simulink model "frft_qpsk_transceiver"  (R2025a)
settings: Solver=FixedStepDiscrete  StartTime=0.0  StopTime=1  RelTol=1e-3
PreLoadFcn:
  | % Add paths
  | addpath("dvb-s2/")
  | addpath("frft_filtering/")
  | addpath("gse")
  | 
  | 
  | 
  | 
  | setTxBurstLength = 10000;
  | txtmsg = ['Zynq radio HW/SW Co-design ÞÞÞÞ']; % Use only printable characters
  | 
  | %------------------------------------------------------------------------------------------------------
  | if ~isequal(size(txtmsg),[1 31])
  |     error('txtmsg must contain 31 characters');
  | end
  | 
  | [dataBits,msg] = zynqRadioHWSWQPSKgenHelloworldMsg(20); % generate 20 msgs for LUT
  | msgLUT = uint8(msg);
  | dataBitsLUT = dataBits(:);
  | Rsym                = 25e3;%1.92e6;
  | Config = zynqRadioHWSWQPSKTxRxParameters;
  | fs = Rsym*Config.SamplesPerSymbol;
  | word = [txtmsg newline];  % append a new line character to txtmsg
  | 
  | % The highest clock rate is 16 times the message character rate.
  | % As the message characters are fed at highest clock to FPGA
  | % repeat each character 16 times to maintain the message rate.
  | word = repelem(word.',16,1);
  | repeatTimes = ceil(setTxBurstLength/length(word));
  | inpData = complex(repmat(uint8(word),repeatTimes,1));
  | inUseTxBurstLength = length(inpData);
PostLoadFcn:
  | hScopeConfig = get_param([gcs '/HDL_QPSK/QPSK Tx Channel QPSK Rx/QPSK Rx/Frequency and Time Synchronizer/Symbol Synchronizer/No HDL/QPSK Receiver Eye Diagram'],'ScopeConfiguration');
  | hScopeConfig.OpenAtSimulationStart = false;
  | hScopeConfig.Visible = false;
  | clear hScopeConfig
InitFcn:
  | setTxBurstLength = 10000;
  | txtmsg = ['Zynq radio HW/SW Co-design ÞÞÞÞ']; % Use only printable characters
  | 
  | %------------------------------------------------------------------------------------------------------
  | if ~isequal(size(txtmsg),[1 31])
  |     error('txtmsg must contain 31 characters');
  | end
  | 
  | [dataBits,msg] = zynqRadioHWSWQPSKgenHelloworldMsg(20); % generate 20 msgs for LUT
  | msgLUT = uint8(msg);
  | dataBitsLUT = dataBits(:);
  | Rsym                = 25e3;%1.92e6;
  | Config = zynqRadioHWSWQPSKTxRxParameters;
  | fs = Rsym*Config.SamplesPerSymbol;
  | word = [txtmsg newline];  % append a new line character to txtmsg
  | 
  | % The highest clock rate is 16 times the message character rate.
  | % As the message characters are fed at highest clock to FPGA
  | % repeat each character 16 times to maintain the message rate.
  | word = repelem(word.',16,1);
  | repeatTimes = ceil(setTxBurstLength/length(word));
  | inpData = complex(repmat(uint8(word),repeatTimes,1));
  | inUseTxBurstLength = length(inpData);
undefined symbols (not defined in the file or in its folder): Add, dspblkCoreblockFVToolHelper, gcbh, Shift, unicode2native
libraries: hdlsllib x120, simulink x39, commseqgen3 x8, dsphdlsigops2 x4, whdledac x4, dsphdlfiltering2 x3, whdlutilities x3, dsphdlxfrm2 x2, dsphdlmathfun2 x2, commdigbbndpm3 x2, commchan3 x1, whdlmod x1
(part 1 of 5)
CloseFcn:
  | clear Config dataBits dataBitsLUT fs h inpData ...
  |         inUseTxBurstLength msg msgLUT repeatTimes ...
  |         Rsym setTxBurstLength simAfterCS simBeforeSS ...
  |         simPeakFind simSyncedPackets simTimingOffset ...
  |         simUserData tout txtmsg word captureASCII
settings Model: DataTypeOverride=Off  SimulationMode=accelerator  Creator=The MathWorks, Inc.  LastModifiedBy=daniel
settings DataIOCC: ReturnWorkspaceOutputs=off
settings OptimizationCC: BlockReduction=off  ConditionallyExecuteInputs=off  DefaultParameterBehavior=Inlined  InheritOutputTypeSmallerThanSingle=on  ReuseModelBlockBuffer=off
settings DebuggingCC: AlgebraicLoopMsg=error  SingleTaskRateTransMsg=error  SubsystemReferenceDiagnosticForUnitTest=warning
settings HardwareCC: ProdBitPerPointer=32.0  ProdBitPerSizeT=32.0  ProdBitPerPtrDiffT=32.0  ProdLargestAtomicFloat=None  ProdIntDivRoundTo=Undefined  ProdEndianess=Unspecified  ProdWordSize=32.0  ProdHWDeviceType=ASIC/FPGA->ASIC/FPGA  TargetBitPerLong=64.0  TargetBitPerPointer=64.0  TargetBitPerSizeT=64.0  TargetBitPerPtrDiffT=64.0  TargetLongLongMode=on  TargetIntDivRoundTo=Zero  TargetEndianess=LittleEndian  TargetWordSize=64.0  TargetHWDeviceType=Custom Processor->MATLAB Host Computer  ProdEqTarget=off
settings RTWCC: GPUComputeCapability=3.5

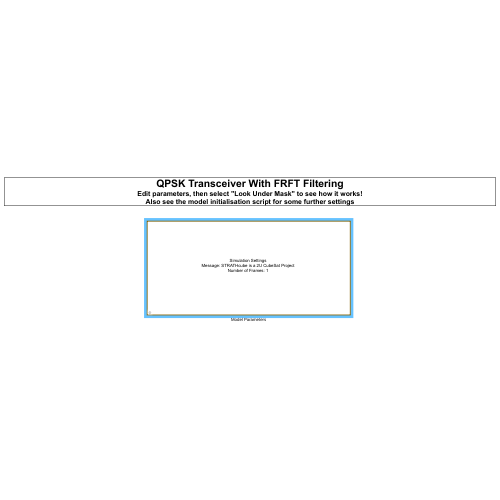
[thumbnail: Simulink's stored preview of the top-level diagram]
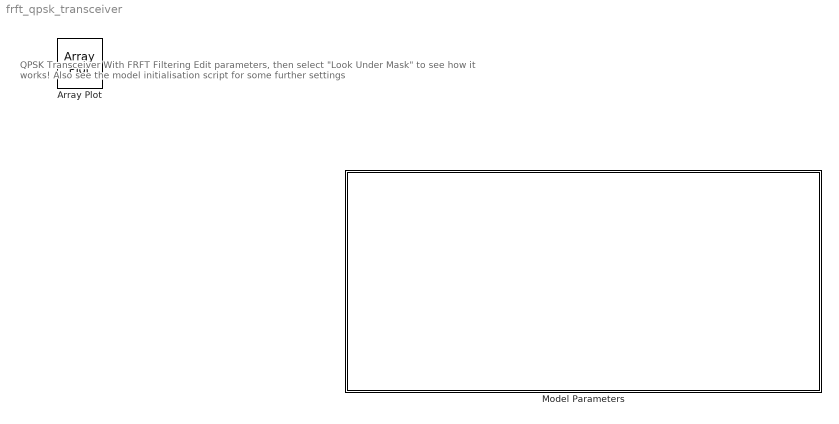
== system frft_qpsk_transceiver ==
  note: QPSK Transceiver With FRFT Filtering
      | Edit parameters, then select "Look Under Mask" to see how it works!
      | Also see the model initialisation script for some further settings
  Model Parameters : Subsystem  mask(Simulation Parameter Controls){fec_en=off, msg="STRATHcube is a 2U CubeSat Project", hmac="SkubeTradeshowDemoKey", n_frames=1, snr=3, interference_en=off, sir=0.1, filter_en=off, altitude=409e3, pass_duration=300, elev_start=10, elev_end=90, fc=435e6}
      mask prompts: fec_en "Enable FEC"; msg "Message Text"; hmac "HMAC Key"; n_frames "N. Frames"; snr "SNR (dB)"; interference_en "Enable Chirp Interference"; sir "SIR (Ratio) (2^n)"; filter_en "Enable Filter"; altitude "Altitude (m)"; pass_duration "Pass Duration (s)"; elev_start "Elevation Start / End (°)"; fc "Carrier Frequency"
      mask help: Sets various parameters for the transceiver system
      mask init:
      | cfg = struct;
      | 
      | % FEC
      | cfg.fec_en = fec_en;
      | gse_frames = gse_genframes(unicode2native(msg),hmac,n_frames)';
      | cfg.FECFRAME = 1120;
      | cfg.DATALENGTH = 840;
      | if fec_en
      |     disp("Using FEC")
      |     
      |     cfg.frames = zeros(cfg.DATALENGTH/8, size(gse_frames,2));
      |     for f = 1:size(gse_frames,2)
      |         frm = gse_frames(:,f);
      |         if length(frm) < cfg.DATALENGTH/8
      |             frm = [frm;zeros(cfg.DATALENGTH/8 - length(frm),1)];
      |         end
      |         cfg.frames(:,f) = frm;
      |     end
      | else
      |     disp("No FEC")
      |     cfg.frames = gse_frames;
      | end
      | 
      | %LDPC Code Setup
      | cfg.parityCheckMatrix =  [5 14 12 1 2 37 45 26 24 0 3 -1 34 7 46 10 -1 -1 -1 -1;
      |     0 35 1 26 0 10 16 16 34 4 2 23 0 51 -1 49 20 -1 -1 -1;
      |     12 28 22 46 3 16 51 2 25 29 19 18 52 -1 37 -1 34 39 -1 -1;
      |     0 51 16 31 13 39 27 33 8 27 53 13 -1 52 33 -1 -1 38 7 -1;
      |     36 6 3 51 4 19 4 45 48 9 -1 11 22 23 43 -1 -1 -1 14 1;];
      | cfg.blockSize = 56;
      | cfg.ipfrms = repelem(cfg.frames(:), 16);
      | 
      | cfg.frame_length = size(cfg.frames,2);
      | cfg.message = msg;
      | cfg.nframes = n_frames;
      | 
      | % Channel
      | cfg.snr = snr; % AWGN
      | 
      | cfg.interference_en = interference_en;
      | cfg.sir = sir;
      | 
      | % Doppler
      | cfg.pass_duration = pass_duration;
      | cfg.doppler_start = dopplerShiftCircularOrbit(elev_start,altitude,10,fc);
      | cfg.doppler_end = dopplerShiftCircularOrbit(elev_end,altitude,10,fc);
      | 
      | cfg.filter_en = filter_en;
      mask DialogControl Container6 Prompt: Transmitter
      mask DialogControl ParameterGroupVar Prompt: GSE Protocol
      mask DialogControl Container3 Prompt: Channel
      mask DialogControl Container4 Prompt: Interference
      mask DialogControl Container5 Prompt: Doppler
      mask Display:
      | icon_txt = sprintf( ...
      |     "Simulation Settings \n" + ...
      |     "Message: %s \n"+ ...
      |     "Number of Frames: %i \n", ...
      |     msg, n_frames ...
      |     );
      | 
      | disp(icon_txt);
  Array Plot : ArrayPlot  IOType=viewer  IsFloating=on  WindowPosition=[560.000000,491.000000,800.000000,500.000000,]  Visible=on  ScopeFrameLocation=window  YLimits=[-203.25 399.25]  DefaultConfigurationName=dsp.scopes.ArrayPlotBlockSpecification

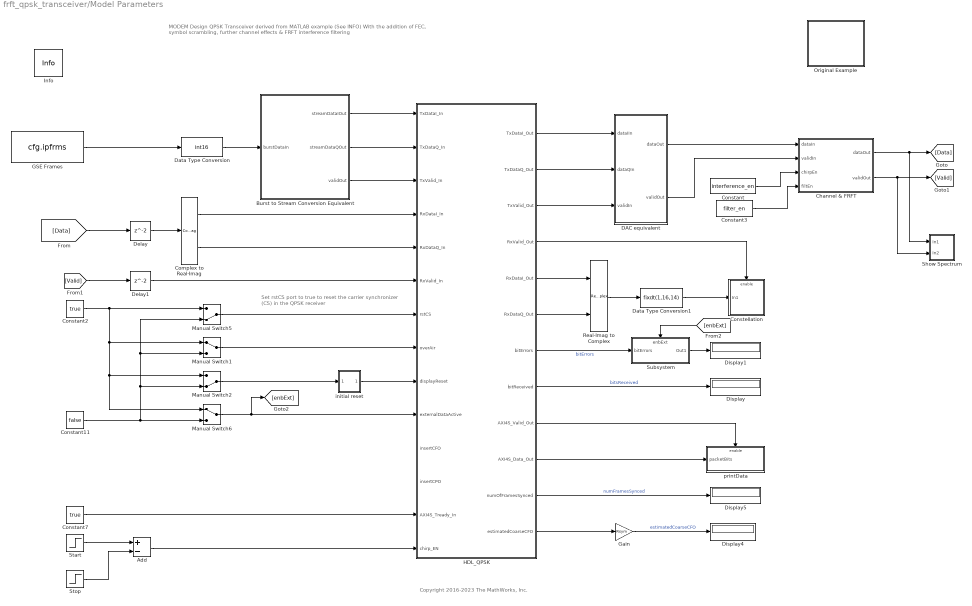
== system frft_qpsk_transceiver/Model Parameters ==
  note: Set rstCS port to true to reset the carrier synchronizer (CS) in the QPSK receiver
  note: Copyright 2016-2023 The MathWorks, Inc.
  note: MODEM Design
      | QPSK Transceiver derived from MATLAB example (See INFO)
      | With the addition of FEC, symbol scrambling, further channel effects & FRFT interference filtering
  Add : Sum  Inputs=+-  OutMin=0  OutMax=1  OutDataTypeStr=fixdt(0,1)
  Burst to Stream Conversion Equivalent : Subsystem
  Channel & FRFT : Subsystem
  Complex to Real-Imag : ComplexToRealImag
  Constant : Constant  Value=interference_en  OutDataTypeStr=boolean
  Constant11 : Constant  Value=false  OutDataTypeStr=boolean  SampleTime=1/fs
  Constant2 : Constant  Value=true  OutDataTypeStr=boolean  SampleTime=1/fs
  Constant3 : Constant  Value=filter_en  OutDataTypeStr=boolean
  Constant7 : Constant  Value=true  OutDataTypeStr=boolean  SampleTime=1/fs
  Constellation : Subsystem
  DAC equivalent : Subsystem
  Data Type Conversion : DataTypeConversion  OutDataTypeStr=int16  SaturateOnIntegerOverflow=off  RndMeth=Floor
  Data Type Conversion1 : DataTypeConversion  OutDataTypeStr=fixdt(1,16,14)  ConvertRealWorld=Stored Integer (SI)  SaturateOnIntegerOverflow=off  RndMeth=Floor
  Delay : Delay
  Delay1 : Delay
  Display{,1,4..5} (4 alike) : Display
  GSE Frames : Constant  Value=cfg.ipfrms  SampleTime=-1
  Gain : Gain  Gain=Rsym  OutDataTypeStr=double
  HDL_QPSK : Subsystem  TreatAsAtomicUnit=on
  Info : sdrzblksprivate/Info  SystemSampleTime=-1  VariantActivationTime=update diagram  EmptyChoice=off  PassThrough=off  PassThroughVariantControl=(default)  EmptyChoiceVariantControl=(default)  AllowFlexibleInterface=on  Latency=0  AutoFrameSizeCalculation=off
  Manual Switch1 : ManualSwitch
  Manual Switch2 : ManualSwitch  CurrentSetting=0
  Manual Switch5 : ManualSwitch  CurrentSetting=0
  Manual Switch6 : ManualSwitch
  Original Example : Subsystem
      settings: OpenFcn="sdrzdoc(\"QPSKTransmitAndReceiveUsingAnalogDevicesAD9361AD9364Example\")"
      mask Display: disp('INFO');
  Real-Imag to Complex : RealImagToComplex
  Show Spectrum : Subsystem
  Start : Step  Time=200e3/fs  SampleTime=1/fs
  Stop : Step  Time=400e3/fs  SampleTime=1/fs
  Subsystem : Subsystem
      settings: PortSchema="{\"entries\":[{\"content\":{\"sides\":[{\"content\":{\"connectorIds\":[\"In1\"]},\"type\":\"ConnectorPlacement.EquallySpacedRectSide\",\"uuid\":\"00e2ba4b-7eac-479c-adca-0b3a47f26300\"},{\"content\":{\"connectorIds\":[\"Out1\"],\"side\":\"RIGHT\"},\"type\":\"ConnectorPlacement.EquallySpacedRectSide\",\"uuid\":\"f46d1850-7aaf-4a4a-a0f0-18f53e4dd1ab\"},{\"content\":{\"connectorIds\":[\"In2\"],\"side\":\"TOP\"},\"type\":\"ConnectorPlacement.EquallySpacedRectSide\",\"uuid\":\"6eb79df9-d0ed-4616-8b56-bf03dd754f89\"}]},\"type\":\"ConnectorPlacement.EquallySpacedConnector\",\"uuid\":\"71623fc3-6fb3-42f9-b5c9-cd74da1aa0dd\"}],\"packageUris\":[\"http://schema.mathworks.com/mf0/Connector/R2020b\"],\"version\":\"1.0\"}"
  initial reset : Subsystem
  printData : Subsystem
  wires:
  initial reset/1(Out1) -> HDL_QPSK/9(displayReset)
  HDL_QPSK/9(AXI4S_Valid_Out) -> printData/Enable
  Burst to Stream Conversion Equivalent/2(streamDataQOut) -> HDL_QPSK/2(TxDataQ_In)
  DAC equivalent/2(validOut) -> Channel & FRFT/2(validIn)
  Add/1 -> HDL_QPSK/14(chirp_EN)
  Constant/1 -> Channel & FRFT/3(chirpEn)
  DAC equivalent/1(dataOut) -> Channel & FRFT/1(dataIn)
  HDL_QPSK/4(RxValid_Out) -> Constellation/Enable
  Start/1 -> Add/1
  Complex to Real-Imag/1 -> HDL_QPSK/4(RxDataI_In)
  HDL_QPSK/8(bitReceived) -> Display/1  "bitsReceived"
  Data Type Conversion/1 -> Burst to Stream Conversion Equivalent/1(burstDataIn)
  Channel & FRFT/1(dataOut) -> Show Spectrum/1(In1), [Data]
  Real-Imag to Complex/1 -> Data Type Conversion1/1
  Subsystem/1(Out1) -> Display1/1
  Constant11/1 -> Manual Switch6/2, Manual Switch5/2, Manual Switch1/2, Manual Switch2/2
  ? -> HDL_QPSK/12(insertCPO)
  [Data] -> Delay/1
  [enbExt] -> Subsystem/2(enbExt)
  Manual Switch1/1 -> HDL_QPSK/8(overAir)
  Data Type Conversion1/1 -> Constellation/1(In1)
  Stop/1 -> Add/2
  Burst to Stream Conversion Equivalent/1(streamDataIOut) -> HDL_QPSK/1(TxDataI_In)
  Constant2/1 -> Manual Switch6/1, Manual Switch2/1, Manual Switch1/1, Manual Switch5/1
  Complex to Real-Imag/2 -> HDL_QPSK/5(RxDataQ_In)
  HDL_QPSK/6(RxDataQ_Out) -> Real-Imag to Complex/2
  HDL_QPSK/1(TxDataI_Out) -> DAC equivalent/1(dataIIn)
  [Valid] -> Delay1/1
  Burst to Stream Conversion Equivalent/3(validOut) -> HDL_QPSK/3(TxValid_In)
  Constant3/1 -> Channel & FRFT/4(filtEn)
  HDL_QPSK/5(RxDataI_Out) -> Real-Imag to Complex/1
  Gain/1 -> Display4/1  "estimatedCoarseCFO"
  Delay1/1 -> HDL_QPSK/6(RxValid_In)
  HDL_QPSK/2(TxDataQ_Out) -> DAC equivalent/2(dataQIn)
  HDL_QPSK/11(numOfFramesSynced) -> Display5/1  "numFramesSynced"
  Manual Switch2/1 -> initial reset/1(In2)
  GSE Frames/1 -> Data Type Conversion/1
  HDL_QPSK/3(TxValid_Out) -> DAC equivalent/3(validIn)
  Constant7/1 -> HDL_QPSK/13(AXI4S_Tready_In)
  HDL_QPSK/10(AXI4S_Data_Out) -> printData/1(packetBits)
  Channel & FRFT/2(validOut) -> Show Spectrum/2(In2), [Valid]
  HDL_QPSK/12(estimatedCoarseCFO) -> Gain/1
  Delay/1 -> Complex to Real-Imag/1
  Manual Switch5/1 -> HDL_QPSK/7(rstCS)
  HDL_QPSK/7(bitErrors) -> Subsystem/1(bitErrors)  "bitErrors"
  Manual Switch6/1 -> HDL_QPSK/10(externalDataActive), [enbExt]

== system frft_qpsk_transceiver/Model Parameters/Burst to Stream Conversion Equivalent ==
  note: The burst data sent from the processing system will be stored in the RAM in the memory channel of SDR IIO radio. The data stored will be poped out as a stream data.
  note: This subsystem does an equivalent operation to simulate the input and output behaviour of the memory channel of the SDR IIO radio.
  burstDataIn : Inport
  Complex to Real-Imag : ComplexToRealImag
  Serializer1D : hdlsllib/HDL Operations/Serializer1D  Ratio=length(cfg.ipfrms)  IdleCycles=0  validIn=off  startOut=off  validOut=on  inputDataDimensions=-1  inputSampleTime=-1  inputSignalType=auto
  streamDataIOut : Outport
  streamDataQOut : Outport  Port=2
  validOut : Outport  Port=3
  wires:
  burstDataIn/1 -> Serializer1D/1
  Serializer1D/1 -> Complex to Real-Imag/1
  Complex to Real-Imag/1 -> streamDataIOut/1
  Complex to Real-Imag/2 -> streamDataQOut/1
  Serializer1D/2 -> validOut/1

== system frft_qpsk_transceiver/Model Parameters/Channel & FRFT ==
  note: Pass through data when chirpEn = 0, otherwise do filtering
  dataIn : Inport
  validIn : Inport  Port=2
  chirpEn : Inport  Port=3
  filtEn : Inport  Port=4
  AWGN : Subsystem
  Data Type Conversion5 : DataTypeConversion  OutDataTypeStr=int16  ConvertRealWorld=Stored Integer (SI)  SaturateOnIntegerOverflow=off  RndMeth=Floor
  Doppler Shift : Subsystem
  Subsystem : Subsystem
  Switch : Switch  Criteria=u2 > Threshold  SaturateOnIntegerOverflow=off  InputSameDT=off
  Switch1 : Switch  Criteria=u2 > Threshold  SaturateOnIntegerOverflow=off  InputSameDT=off
  add_chirp : MATLAB Function  TreatAsAtomicUnit=on  mask{fs=fs, T=32e-3, f0=0, f1=0.9*fs/2, sir=sir}
      mask prompts: sir "SIR (Ratio)"
  dataOut : Outport
      settings: SignalType=complex
  validOut : Outport  Port=2
  wires:
  Switch1/1 -> validOut/1
  chirpEn/1 -> add_chirp/3(chirpEn)
  add_chirp/1(sigOut) -> Switch/3, Subsystem/1(sigIn)  "chirp_sig"
  add_chirp/2(validOut) -> Switch1/3, Subsystem/2(validIn)
  filtEn/1 -> Switch1/2, Switch/2
  Subsystem/2(ValidOut) -> Switch1/1
  Subsystem/1(S) -> Switch/1
  Switch/1 -> Data Type Conversion5/1
  Data Type Conversion5/1 -> dataOut/1
  dataIn/1 -> Doppler Shift/1(dataIn)
  validIn/1 -> Doppler Shift/2(validIn)
  Doppler Shift/1(Out1) -> AWGN/1(dataIn)
  Doppler Shift/2(Out2) -> AWGN/2(validIn)
  AWGN/1(dataOut) -> add_chirp/1(sigIn)
  AWGN/2(validOut) -> add_chirp/2(validIn)

== system frft_qpsk_transceiver/Model Parameters/Constellation ==
  In1 : Inport
  Enable : EnablePort
  Constellation Diagram : ConstellationDiagram  WindowPosition=[1388.000000,624.000000,653.000000,531.000000,]  Visible=on  ScopeFrameLocation=window  SymbolsToDisplaySource=Property  SymbolsToDisplay=10000  XLimits=[-1.38,1.38]  YLimits=[-1.38,1.38]  AxesLimits=[-1.38,1.38]  DefaultConfigurationName=comm.scopes.ConstellationDiagramBlockCfg
  Terminator : Terminator
  wires:
  In1/1 -> Constellation Diagram/1, Terminator/1

== system frft_qpsk_transceiver/Model Parameters/DAC equivalent ==
  dataIIn : Inport
  dataQIn : Inport  Port=2
  validIn : Inport  Port=3
  Data Type Conversion : DataTypeConversion  OutDataTypeStr=int16  SaturateOnIntegerOverflow=off  RndMeth=Floor
  Extract Bits : simulink/Logic and Bit Operations/Extract Bits  bitsToExtract=Range starting with most significant bit  numBits=12  bitIdxRange=[0 7]  outScalingMode=Treat bit field as an integer
  Extract Bits1 : simulink/Logic and Bit Operations/Extract Bits  bitsToExtract=Range starting with most significant bit  numBits=12  bitIdxRange=[0 7]  outScalingMode=Treat bit field as an integer
  Real-Imag to Complex : RealImagToComplex
  dataOut : Outport
  validOut : Outport  Port=2
  wires:
  dataIIn/1 -> Extract Bits/1
  dataQIn/1 -> Extract Bits1/1
  Extract Bits/1 -> Real-Imag to Complex/1
  Extract Bits1/1 -> Real-Imag to Complex/2
  Real-Imag to Complex/1 -> Data Type Conversion/1
  validIn/1 -> validOut/1
  Data Type Conversion/1 -> dataOut/1

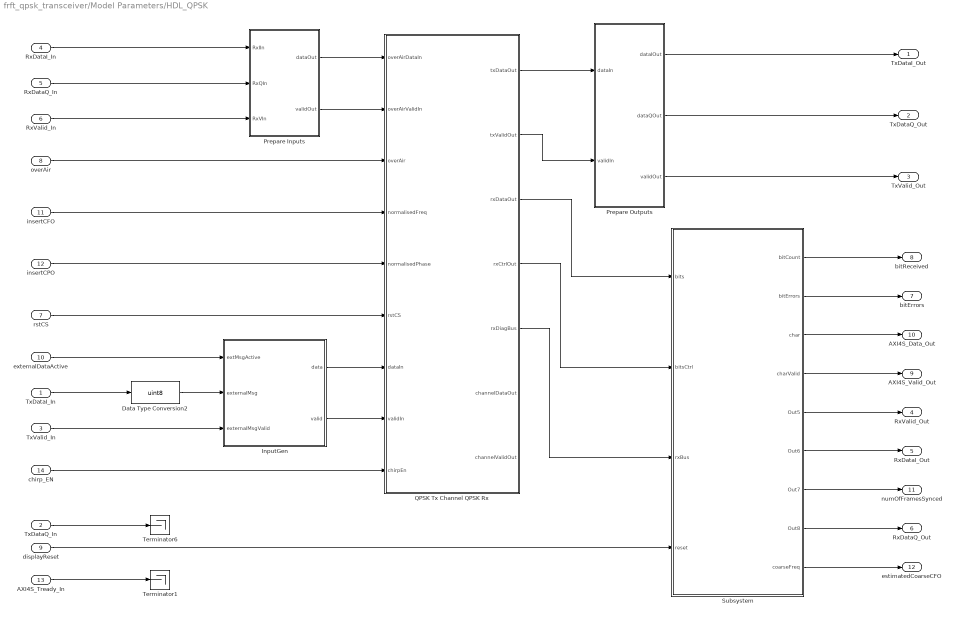
== system frft_qpsk_transceiver/Model Parameters/HDL_QPSK ==
  TxDataI_In : Inport
  TxDataQ_In : Inport  Port=2
  TxValid_In : Inport  Port=3
  RxDataI_In : Inport  Port=4
  RxDataQ_In : Inport  Port=5
  RxValid_In : Inport  Port=6
  rstCS : Inport  Port=7
  overAir : Inport  Port=8
  displayReset : Inport  Port=9
  externalDataActive : Inport  Port=10
  insertCFO : Inport  Port=11
  insertCPO : Inport  Port=12
  AXI4S_Tready_In : Inport  Port=13
  chirp_EN : Inport  Port=14
  Data Type Conversion2 : DataTypeConversion  OutDataTypeStr=uint8  SaturateOnIntegerOverflow=off  RndMeth=Floor
  InputGen : Subsystem
  Prepare Inputs : Subsystem
  Prepare Outputs : Subsystem
  QPSK Tx Channel QPSK Rx : Subsystem
  Subsystem : Subsystem
  Terminator1 : Terminator
  Terminator6 : Terminator
  TxDataI_Out : Outport
  TxDataQ_Out : Outport  Port=2
  TxValid_Out : Outport  Port=3
  RxValid_Out : Outport  Port=4
  RxDataI_Out : Outport  Port=5
  RxDataQ_Out : Outport  Port=6
  bitErrors : Outport  Port=7
  bitReceived : Outport  Port=8
  AXI4S_Valid_Out : Outport  Port=9
  AXI4S_Data_Out : Outport  Port=10
  numOfFramesSynced : Outport  Port=11
  estimatedCoarseCFO : Outport  Port=12
  wires:
  Prepare Outputs/2(dataQOut) -> TxDataQ_Out/1
  Prepare Outputs/3(validOut) -> TxValid_Out/1
  AXI4S_Tready_In/1 -> Terminator1/1
  Prepare Inputs/1(dataOut) -> QPSK Tx Channel QPSK Rx/1(overAirDataIn)
  Prepare Inputs/2(validOut) -> QPSK Tx Channel QPSK Rx/2(overAirValidIn)
  InputGen/1(data) -> QPSK Tx Channel QPSK Rx/7(dataIn)
  InputGen/2(valid) -> QPSK Tx Channel QPSK Rx/8(validIn)
  overAir/1 -> QPSK Tx Channel QPSK Rx/3(overAir)
  insertCFO/1 -> QPSK Tx Channel QPSK Rx/4(normalisedFreq)
  insertCPO/1 -> QPSK Tx Channel QPSK Rx/5(normalisedPhase)
  QPSK Tx Channel QPSK Rx/1(txDataOut) -> Prepare Outputs/1(dataIn)
  QPSK Tx Channel QPSK Rx/2(txValidOut) -> Prepare Outputs/2(validIn)
  displayReset/1 -> Subsystem/4(reset)
  QPSK Tx Channel QPSK Rx/3(rxDataOut) -> Subsystem/1(bits)
  QPSK Tx Channel QPSK Rx/4(rxCtrlOut) -> Subsystem/2(bitsCtrl)
  QPSK Tx Channel QPSK Rx/5(rxDiagBus) -> Subsystem/3(rxBus)
  Subsystem/1(bitCount) -> bitReceived/1
  Subsystem/2(bitErrors) -> bitErrors/1
  Subsystem/3(char) -> AXI4S_Data_Out/1
  Subsystem/4(charValid) -> AXI4S_Valid_Out/1
  Subsystem/5(Out5) -> RxValid_Out/1
  Subsystem/6(Out6) -> RxDataI_Out/1
  Subsystem/7(Out7) -> numOfFramesSynced/1
  Subsystem/8(Out8) -> RxDataQ_Out/1
  rstCS/1 -> QPSK Tx Channel QPSK Rx/6(rstCS)
  Subsystem/9(coarseFreq) -> estimatedCoarseCFO/1
  Prepare Outputs/1(dataIOut) -> TxDataI_Out/1
  RxDataI_In/1 -> Prepare Inputs/1(RxIIn)
  RxDataQ_In/1 -> Prepare Inputs/2(RxQIn)
  RxValid_In/1 -> Prepare Inputs/3(RxVIn)
  TxValid_In/1 -> InputGen/3(externalMsgValid)
  TxDataQ_In/1 -> Terminator6/1
  externalDataActive/1 -> InputGen/1(extMsgActive)
  TxDataI_In/1 -> Data Type Conversion2/1
  Data Type Conversion2/1 -> InputGen/2(externalMsg)
  chirp_EN/1 -> QPSK Tx Channel QPSK Rx/9(chirpEn)

== system frft_qpsk_transceiver/Model Parameters/Original Example ==

== system frft_qpsk_transceiver/Model Parameters/Show Spectrum ==
  In1 : Inport
  In2 : Inport  Port=2
  Compare To Constant : simulink/Logic and Bit Operations/Compare To Constant  relop===  const=inf  OutDataTypeStr=boolean
  Compare To Constant1 : simulink/Logic and Bit Operations/Compare To Constant  relop===  const=NaN  OutDataTypeStr=boolean
  Constant1 : Constant  Value=complex(0+0i)
  Data Type Conversion5 : DataTypeConversion  OutDataTypeStr=double  ConvertRealWorld=Stored Integer (SI)  SaturateOnIntegerOverflow=off  RndMeth=Floor
  Delay2 : Delay  DelayLength=1
  Delay3 : Delay  DelayLength=1
  OR : Logic  Operator=OR  IconShape=distinctive  AllPortsSameDT=off  OutDataTypeStr=boolean
  Spectrum Analyzer : SpectrumAnalyzer  WindowPosition=[511.000000,647.000000,1440.000000,699.000000,]  Visible=on  ScopeFrameLocation=window  ViewType=Spectrum and spectrogram  WindowInvariantSamplesPerUpdate=on  Span=160000  StartFrequency=-80000  StopFrequency=80000  YLimits=[-22.703734811580006 91.64033184798589]  ColorLimits=[NaN NaN]
  Switch : Switch  Criteria=u2 > Threshold  OutDataTypeStr=Inherit: Inherit via back propagation  SaturateOnIntegerOverflow=off
  Switch1 : Switch  Criteria=u2 > Threshold  OutDataTypeStr=Inherit: Inherit via back propagation  SaturateOnIntegerOverflow=off
  wires:
  Delay2/1 -> Delay3/1
  Compare To Constant/1 -> OR/1
  Constant1/1 -> Switch1/1, Switch/3
  Delay3/1 -> Switch1/3
  Data Type Conversion5/1 -> Switch/1
  Switch/1 -> Delay2/1, Compare To Constant1/1, Compare To Constant/1
  Switch1/1 -> Spectrum Analyzer/1
  OR/1 -> Switch1/2
  In2/1 -> Switch/2
  Compare To Constant1/1 -> OR/2
  In1/1 -> Data Type Conversion5/1

== system frft_qpsk_transceiver/Model Parameters/Subsystem ==
  note: 2^32-1 will be treated as NaN in double when converted to double
  bitErrors : Inport
  enbExt : Inport  Port=2
  Compare To Constant : simulink/Logic and Bit Operations/Compare To Constant  relop===  const=2^32-1  OutDataTypeStr=boolean
  Constant : Constant  Value=2^32-1  OutDataTypeStr=uint32  SampleTime=-1
  Constant1 : Constant  Value=NaN  SampleTime=-1
  Data Type Conversion3 : DataTypeConversion  OutDataTypeStr=double  SaturateOnIntegerOverflow=off  RndMeth=Floor
  Switch : Switch  Criteria=u2 ~= 0  SaturateOnIntegerOverflow=off  InputSameDT=off
  Switch1 : Switch  Criteria=u2 ~= 0  SaturateOnIntegerOverflow=off  InputSameDT=off
  Out1 : Outport
  wires:
  Constant/1 -> Switch/1
  bitErrors/1 -> Switch/3
  enbExt/1 -> Switch/2
  Compare To Constant/1 -> Switch1/2
  Switch1/1 -> Out1/1
  Switch/1 -> Data Type Conversion3/1, Compare To Constant/1
  Data Type Conversion3/1 -> Switch1/3
  Constant1/1 -> Switch1/1

== system frft_qpsk_transceiver/Model Parameters/initial reset ==
  In2 : Inport
  Constant : Constant  OutDataTypeStr=boolean  SampleTime=-1
  Delay : Delay  DelayLength=1
  Logical Operator : Logic  Operator=OR  IconShape=distinctive  AllPortsSameDT=off  OutDataTypeStr=boolean
  Logical Operator1 : Logic  Operator=XOR  IconShape=distinctive  AllPortsSameDT=off  OutDataTypeStr=boolean
  Out1 : Outport
  wires:
  In2/1 -> Logical Operator/2
  Logical Operator1/1 -> Logical Operator/1
  Logical Operator/1 -> Out1/1
  Constant/1 -> Delay/1, Logical Operator1/1
  Delay/1 -> Logical Operator1/2

== system frft_qpsk_transceiver/Model Parameters/printData ==
  packetBits : Inport
  Enable : EnablePort  PropagateVarSize=During execution
  Extract Bits : simulink/Logic and Bit Operations/Extract Bits  bitsToExtract=Range ending with least significant bit  numBits=8  bitIdxRange=[0 7]  outScalingMode=Treat bit field as an integer
  Extract Bits1 : simulink/Logic and Bit Operations/Extract Bits  bitsToExtract=Range of bits  numBits=8  bitIdxRange=[8,8]  outScalingMode=Treat bit field as an integer
  Extract Bits2 : simulink/Logic and Bit Operations/Extract Bits  bitsToExtract=Range of bits  numBits=8  bitIdxRange=[9,9]  outScalingMode=Treat bit field as an integer
  MATLAB Function : MATLAB Function  TreatAsAtomicUnit=on  mask{msg_length=size(cfg.frames,1)  - 9 - 32+1, frame_length=size(cfg.frames,1), msg_orig=unicode2native(msg)}
      mask prompts: msg_length "Message Length"; frame_length "Frame Length"; msg_orig "Original Message"
  RxFrame : ToWorkspace  VariableName=RxFrame  SaveFormat=Structure  SampleTime=-1
      settings: Save2DSignal=2-D array (concatenate along first dimension)
  RxFrameValid : ToWorkspace  VariableName=RxFrameValid  SampleTime=-1
      settings: Save2DSignal=2-D array (concatenate along first dimension)
  Serializer1D : hdlsllib/HDL Operations/Serializer1D  Ratio=1  IdleCycles=0  validIn=off  startOut=off  validOut=off  inputDataDimensions=-1  inputSampleTime=-1  inputSignalType=auto
  captureASCII : ToWorkspace  VariableName=captureASCII  SampleTime=-1
      settings: Save2DSignal=2-D array (concatenate along first dimension)
  wires:
  packetBits/1 -> Serializer1D/1
  Serializer1D/1 -> Extract Bits/1, Extract Bits1/1, Extract Bits2/1
  Extract Bits/1 -> MATLAB Function/3(u), captureASCII/1
  Extract Bits2/1 -> MATLAB Function/1(frm_start)
  Extract Bits1/1 -> MATLAB Function/2(frm_end)
  MATLAB Function/1(frameOut) -> RxFrame/1
  MATLAB Function/2(frameValid) -> RxFrameValid/1

== system frft_qpsk_transceiver/Model Parameters/Channel & FRFT/AWGN ==
  dataIn : Inport
  validIn : Inport  Port=2
  AWGN Channel : commchan3/AWGN Channel  LegacyMode=off  NoiseMethod="Signal to noise ratio  (SNR)"  noiseMode="Signal to noise ratio  (SNR)"  EbNo=10  EsNo=10  SNR=cfg.snr-30  BitsPerSymbol=1  SignalPower=1  SpecifySymbolPeriod=off  SamplesPerSymbol=1  SymbolPeriod=1  VarianceSource=Parameter  Variance=1  RandomStream=Global stream  Seed=67  SimulateUsing=Code generation
  Cast : DataTypeConversion  SaturateOnIntegerOverflow=off  RndMeth=Floor
  Delay : Delay  DelayLength=1
  dataOut : Outport
  validOut : Outport  Port=2
  wires:
  Cast/1 -> AWGN Channel/1
  dataIn/1 -> Cast/1  "awgn_in"
  Delay/1 -> validOut/1
  AWGN Channel/1 -> dataOut/1  "awgn_out"
  validIn/1 -> Delay/1

== system frft_qpsk_transceiver/Model Parameters/Channel & FRFT/Doppler Shift ==
  dataIn : Inport
  validIn : Inport  Port=2
  CPO : Constant  Value=fi(phase,1,21,21)  SampleTime=1/fs  mask{phased=0}
      mask prompts: phased "CPO (degrees):"
      mask init:
      | phase = phased/360;
      mask DialogControl DescGroupVar Prompt: Insert CPO
      mask DialogControl DescTextVar Prompt: Introduce CPO into transmitter waveform. The overAir port must be set to false. CPO range: -180 to less than 180
      mask Display: disp(get_param(gcb,"phased"));
  Data Type Conversion : DataTypeConversion  OutDataTypeStr=fixdt(1,21,0)  ConvertRealWorld=Stored Integer (SI)  SaturateOnIntegerOverflow=off  RndMeth=Floor
  Data Type Conversion1 : DataTypeConversion  OutDataTypeStr=fixdt(1,21,0)  ConvertRealWorld=Stored Integer (SI)  SaturateOnIntegerOverflow=off  RndMeth=Floor
  Delay : Delay  DelayLength=6
  Doppler Shift : Sin  SineType=Sample based  Amplitude=-cfg.doppler_start  Frequency=2*pi  Phase=pi  Samples=cfg.pass_duration*fs  SampleTime=1/fs
  NCO HDL Optimized : dsphdlsigops2/NCO  PhaseIncrementSource=Input port  PhaseIncrement=100  PhaseOffsetSource=Input port  PhaseOffset=0  DitherSource=Property  NumDitherBits=11  SamplesPerFrame=1  LUTCompress=off  ResetAction=off  Waveform=Complex exponential  PhasePort=off  SimulateUsing=Code generation  AccumulatorWL=21  PhaseQuantization=on  NumQuantizerAccumulatorBits=14  OutputDataType=Binary point scaling  OutputWL=16  OutputFL=14
  Product : Product  OutDataTypeStr=Inherit: Same as first input
  Out1 : Outport
  Out2 : Outport  Port=2
  wires:
  dataIn/1 -> Delay/1
  Delay/1 -> Product/1
  Data Type Conversion/1 -> NCO HDL Optimized/1
  NCO HDL Optimized/1 -> Product/2
  Product/1 -> Out1/1
  Data Type Conversion1/1 -> NCO HDL Optimized/2
  Doppler Shift/1 -> Data Type Conversion/1
  NCO HDL Optimized/2 -> Out2/1
  CPO/1 -> Data Type Conversion1/1
  validIn/1 -> NCO HDL Optimized/3

== system frft_qpsk_transceiver/Model Parameters/Channel & FRFT/Subsystem ==
  note: x = FRFT( FRFT(x, a), -a )
  sigIn : Inport
  validIn : Inport  Port=2
  Gain : Gain  Gain=-1
  Parallel2Serial : hdlsllib/HDL Operations/Serializer1D  Ratio=4000  IdleCycles=0  validIn=on  startOut=off  validOut=on  inputDataDimensions=-1  inputSampleTime=-1  inputSignalType=complex
  Serial2Parallel : hdlsllib/HDL Operations/Deserializer1D  Ratio=4000  IdleCycles=0  InitialCondition=0  startIn=off  validIn=on  validOut=on  inputDataDimensions=-1  inputSampleTime=-1  inputSignalType=auto
  frft_filter : MATLAB Function  TreatAsAtomicUnit=on  mask{thresh=2e3}
      mask prompts: thresh "Peak Threshold"
  frft_peaksearch : MATLAB Function  TreatAsAtomicUnit=on  mask{n_iterations=100, p_low=0, p_high=2}
      mask prompts: n_iterations "Number of Iterations"; p_low "Low"; p_high "High"
  frft_transform : MATLAB Function  TreatAsAtomicUnit=on  mask{n_iterations=100, p_low=0.5, p_high=1.5}
      mask prompts: n_iterations "Number of Iterations"; p_low "Low"; p_high "High"
  windowing : MATLAB Function  TreatAsAtomicUnit=on  mask{gamma=0.9}
      mask prompts: gamma "Γ"
  S : Outport
  ValidOut : Outport  Port=2
  wires:
  frft_peaksearch/3(p_max) -> Gain/1  "frft_p"
  validIn/1 -> Serial2Parallel/2
  frft_transform/1(sigOut) -> Parallel2Serial/1  "ifrft_sig"
  Parallel2Serial/2 -> ValidOut/1
  Parallel2Serial/1 -> S/1  "ifrft_sig"
  frft_filter/2(validOut) -> frft_transform/2(validIn)
  frft_transform/2(validOut) -> Parallel2Serial/2
  frft_peaksearch/2(validOut) -> frft_filter/2(validIn)
  frft_peaksearch/1(sigOut) -> frft_filter/1(sigIn)  "frft_sig"
  Gain/1 -> frft_transform/3(p)
  frft_filter/1(sigOut) -> frft_transform/1(sigIn)  "frft_filt"
  sigIn/1 -> Serial2Parallel/1
  Serial2Parallel/1 -> windowing/1(sigIn)
  Serial2Parallel/2 -> windowing/2(validIn)
  windowing/1(sigOut) -> frft_peaksearch/1(sigIn)  "frft_sig"
  windowing/2(validOut) -> frft_peaksearch/2(validIn)

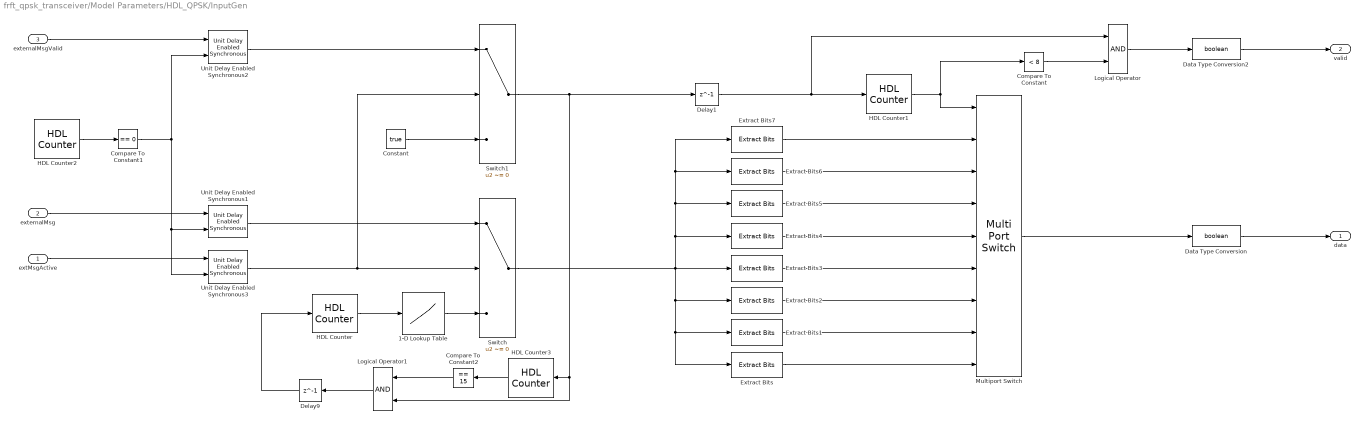
== system frft_qpsk_transceiver/Model Parameters/HDL_QPSK/InputGen ==
  extMsgActive : Inport
  externalMsg : Inport  Port=2
  externalMsgValid : Inport  Port=3
  1-D Lookup Table : Lookup_n-D  NumberOfTableDimensions=1  LookupTableObject=''  BreakpointsForDimension1=0:length(msgLUT) - 1  BreakpointsForDimension1FirstPoint=10  BreakpointsForDimension2FirstPoint=10  BreakpointsForDimension1Spacing=12  BreakpointsForDimension2Spacing=12  IndexSearchMethod=Evenly spaced points  Table=msgLUT  TableDataTypeStr=uint8  InterpMethod=Flat  DiagnosticForOutOfRangeInput=Error  InternalRulePriority=Speed  OutDataTypeStr=uint8  RndMeth=Simplest
  Compare To Constant : simulink/Logic and Bit Operations/Compare To Constant  relop=<  const=8  OutDataTypeStr=boolean
  Compare To Constant1 : hdlsllib/Logic and Bit Operations/Compare To Constant  relop===  const=0  OutDataTypeStr=boolean
  Compare To Constant2 : hdlsllib/Logic and Bit Operations/Compare To Constant  relop===  const=15  OutDataTypeStr=boolean
  Constant : Constant  Value=true  SampleTime=-1
  Data Type Conversion : DataTypeConversion  OutDataTypeStr=boolean  SaturateOnIntegerOverflow=off  RndMeth=Floor
  Data Type Conversion2 : DataTypeConversion  OutDataTypeStr=boolean  SaturateOnIntegerOverflow=off  RndMeth=Floor
  Delay1 : Delay  DelayLength=1
  Delay9 : Delay  DelayLength=1
  Extract Bits : simulink/Logic and Bit Operations/Extract Bits  bitsToExtract=Range of bits  numBits=8  bitIdxRange=0  outScalingMode=Treat bit field as an integer
  Extract Bits1 : simulink/Logic and Bit Operations/Extract Bits  bitsToExtract=Range of bits  numBits=8  bitIdxRange=1  outScalingMode=Treat bit field as an integer
  Extract Bits2 : simulink/Logic and Bit Operations/Extract Bits  bitsToExtract=Range of bits  numBits=8  bitIdxRange=2  outScalingMode=Treat bit field as an integer
  Extract Bits3 : simulink/Logic and Bit Operations/Extract Bits  bitsToExtract=Range of bits  numBits=8  bitIdxRange=3  outScalingMode=Treat bit field as an integer
  Extract Bits4 : simulink/Logic and Bit Operations/Extract Bits  bitsToExtract=Range of bits  numBits=8  bitIdxRange=4  outScalingMode=Treat bit field as an integer
  Extract Bits5 : simulink/Logic and Bit Operations/Extract Bits  bitsToExtract=Range of bits  numBits=8  bitIdxRange=5  outScalingMode=Treat bit field as an integer
  Extract Bits6 : simulink/Logic and Bit Operations/Extract Bits  bitsToExtract=Range of bits  numBits=8  bitIdxRange=6  outScalingMode=Treat bit field as an integer
  Extract Bits7 : simulink/Logic and Bit Operations/Extract Bits  bitsToExtract=Range of bits  numBits=8  bitIdxRange=7  outScalingMode=Treat bit field as an integer
  HDL Counter : hdlsllib/Sources/HDL Counter  CountType=Count limited  CountInit=0  CountStep=1  CountMax=length(msgLUT) - 1  CountFromType=Initial value  CountFrom=0  CountResetPort=off  CountLoadPort=off  CountEnbPort=on  CountDirPort=off  CountHitOutputPort=off  CountDataType=Unsigned  CountWordLen=nextpow2(length(msgLUT) - 1)  CountFracLen=0  CountSampTime=8/(Rsym*2)
  HDL Counter1 : hdlsllib/Sources/HDL Counter  CountType=Count limited  CountInit=0  CountStep=1  CountMax=15  CountFromType=Initial value  CountFrom=0  CountResetPort=off  CountLoadPort=off  CountEnbPort=on  CountDirPort=off  CountHitOutputPort=off  CountDataType=Unsigned  CountWordLen=4  CountFracLen=0  CountSampTime=1
  HDL Counter2 : hdlsllib/Sources/HDL Counter  CountType=Count limited  CountInit=0  CountStep=1  CountMax=15  CountFromType=Initial value  CountFrom=0  CountResetPort=off  CountLoadPort=off  CountEnbPort=off  CountDirPort=off  CountHitOutputPort=off  CountDataType=Unsigned  CountWordLen=4  CountFracLen=0  CountSampTime=1/fs
  HDL Counter3 : hdlsllib/Sources/HDL Counter  CountType=Count limited  CountInit=0  CountStep=1  CountMax=15  CountFromType=Initial value  CountFrom=0  CountResetPort=off  CountLoadPort=off  CountEnbPort=on  CountDirPort=off  CountHitOutputPort=off  CountDataType=Unsigned  CountWordLen=4  CountFracLen=0  CountSampTime=1/fs
  Logical Operator : Logic  AllPortsSameDT=off  OutDataTypeStr=boolean
  Logical Operator1 : Logic  AllPortsSameDT=off  OutDataTypeStr=boolean
  Multiport Switch : MultiPortSwitch  DataPortOrder=Zero-based contiguous  Inputs=8  DiagnosticForDefault=None  zeroidx=on  SaturateOnIntegerOverflow=off  InputSameDT=off
  Switch : Switch  Criteria=u2 ~= 0  SaturateOnIntegerOverflow=off  InputSameDT=off
  Switch1 : Switch  Criteria=u2 ~= 0  SaturateOnIntegerOverflow=off  InputSameDT=off
  Unit Delay Enabled Synchronous1 : hdlsllib/Discrete/Unit Delay Enabled Synchronous  InitialCondition=0.0  SampleTime=-1
  Unit Delay Enabled Synchronous2 : hdlsllib/Discrete/Unit Delay Enabled Synchronous  InitialCondition=0.0  SampleTime=-1
  Unit Delay Enabled Synchronous3 : hdlsllib/Discrete/Unit Delay Enabled Synchronous  InitialCondition=0.0  SampleTime=-1
  data : Outport
  valid : Outport  Port=2
  wires:
  Logical Operator1/1 -> Delay9/1
  Unit Delay Enabled Synchronous2/1 -> Switch1/1
  Multiport Switch/1 -> Data Type Conversion/1
  Unit Delay Enabled Synchronous1/1 -> Switch/1
  Extract Bits/1 -> Multiport Switch/9
  Extract Bits1/1 -> Multiport Switch/8
  HDL Counter1/1 -> Multiport Switch/1, Compare To Constant/1
  HDL Counter/1 -> 1-D Lookup Table/1
  1-D Lookup Table/1 -> Switch/3
  externalMsgValid/1 -> Unit Delay Enabled Synchronous2/1
  Logical Operator/1 -> Data Type Conversion2/1
  Data Type Conversion2/1 -> valid/1
  Delay9/1 -> HDL Counter/1
  Extract Bits2/1 -> Multiport Switch/7
  Extract Bits3/1 -> Multiport Switch/6
  Compare To Constant2/1 -> Logical Operator1/1
  Unit Delay Enabled Synchronous3/1 -> Switch/2, Switch1/2
  Extract Bits5/1 -> Multiport Switch/4
  Extract Bits4/1 -> Multiport Switch/5
  externalMsg/1 -> Unit Delay Enabled Synchronous1/1
  Delay1/1 -> Logical Operator/1, HDL Counter1/1
  Switch/1 -> Extract Bits6/1, Extract Bits7/1, Extract Bits5/1, Extract Bits4/1, Extract Bits2/1, Extract Bits1/1, Extract Bits/1, Extract Bits3/1
  Data Type Conversion/1 -> data/1
  Compare To Constant1/1 -> Unit Delay Enabled Synchronous1/2, Unit Delay Enabled Synchronous3/2, Unit Delay Enabled Synchronous2/2
  HDL Counter3/1 -> Compare To Constant2/1
  Extract Bits6/1 -> Multiport Switch/3
  Switch1/1 -> Delay1/1, HDL Counter3/1, Logical Operator1/2
  Constant/1 -> Switch1/3
  Compare To Constant/1 -> Logical Operator/2
  HDL Counter2/1 -> Compare To Constant1/1
  extMsgActive/1 -> Unit Delay Enabled Synchronous3/1
  Extract Bits7/1 -> Multiport Switch/2

== system frft_qpsk_transceiver/Model Parameters/HDL_QPSK/Prepare Inputs ==
  RxIIn : Inport
  RxQIn : Inport  Port=2
  RxVIn : Inport  Port=3
  Data Type Conversion5 : DataTypeConversion  OutDataTypeStr=fixdt(1,16,14)  ConvertRealWorld=Stored Integer (SI)  SaturateOnIntegerOverflow=off  RndMeth=Floor
  Delay{1,3..4,6} (4 alike) : Delay
  Delay2 : Delay  DelayLength=4
  Delay5 : Delay  DelayLength=4
  Gain : Gain  Gain=16  ParamDataTypeStr=fixdt(0,5,0)  OutDataTypeStr=Inherit: Same as input
  Real-Imag to Complex : RealImagToComplex
  dataOut : Outport
  validOut : Outport  Port=2
  wires:
  RxIIn/1 -> Real-Imag to Complex/1
  Gain/1 -> Delay2/1
  Real-Imag to Complex/1 -> Data Type Conversion5/1
  Delay5/1 -> Delay6/1
  Data Type Conversion5/1 -> Delay1/1
  Delay2/1 -> Delay3/1
  Delay4/1 -> Delay5/1
  RxQIn/1 -> Real-Imag to Complex/2
  Delay1/1 -> Gain/1
  RxVIn/1 -> Delay4/1
  Delay6/1 -> validOut/1
  Delay3/1 -> dataOut/1

== system frft_qpsk_transceiver/Model Parameters/HDL_QPSK/Prepare Outputs ==
  dataIn : Inport
  validIn : Inport  Port=2
  Complex to Real-Imag1 : ComplexToRealImag
  Data Type Conversion4 : DataTypeConversion  OutDataTypeStr=int16  ConvertRealWorld=Stored Integer (SI)  SaturateOnIntegerOverflow=off  RndMeth=Floor
  Delay7 : Delay
  Delay8 : Delay
  Delay9 : Delay
  dataIOut : Outport
  dataQOut : Outport  Port=2
  validOut : Outport  Port=3
  wires:
  dataIn/1 -> Data Type Conversion4/1
  Delay7/1 -> dataIOut/1
  Complex to Real-Imag1/2 -> Delay8/1
  validIn/1 -> Delay9/1
  Complex to Real-Imag1/1 -> Delay7/1
  Data Type Conversion4/1 -> Complex to Real-Imag1/1
  Delay9/1 -> validOut/1
  Delay8/1 -> dataQOut/1

== system frft_qpsk_transceiver/Model Parameters/HDL_QPSK/QPSK Tx Channel QPSK Rx ==
  overAirDataIn : Inport
  overAirValidIn : Inport  Port=2
  overAir : Inport  Port=3
  normalisedFreq : Inport  Port=4
  normalisedPhase : Inport  Port=5
  rstCS : Inport  Port=6
  dataIn : Inport  Port=7
  validIn : Inport  Port=8
  chirpEn : Inport  Port=9
  Data Type Conversion7 : DataTypeConversion  OutDataTypeStr=fixdt(1,16,14)  SaturateOnIntegerOverflow=off  RndMeth=Floor
  QPSK Rx : Subsystem  mask{rawlen=size(cfg.frames,1)*8, fec_en=cfg.fec_en, FECFRAME=cfg.FECFRAME}
      mask prompts: rawlen "No. Data Bits in Frame"; fec_en "FEC Enabled"; FECFRAME "FECFRAME Length"
      mask init:
      | integAvgLen = 2^15;
      | 
      | RxParams            = zynqRadioHWSWQPSKTxRxParameters();
      | Preamble            = RxParams.Preamble;
      | QPSKConstellation   = RxParams.QPSKConstellation;
      | 
      | if fec_en
      |     dataBits = FECFRAME;
      | else
      |     dataBits = rawlen;
      | end
      | 
      | dataBitsPerPacket   = dataBits;
      | 
      | 
      | SamplesPerSymbol    = RxParams.SamplesPerSymbol;
      | RRCCoef             = RxParams.RRCCoef;
      | bitsPerPacket        = dataBitsPerPacket + length(Preamble);
      | 
      | rxPreambleMFCoeffs  = RxParams.rxPreambleMFCoeffs;
      | preambleSymbols     = RxParams.preambleSymbols;
      | ThresoldGainFac     = RxParams.ThresoldGainFac;
      | 
      | % AGC Parameters
      | AGCReference           = RxParams.AGCReference;
      | AGCLoopGain            = RxParams.AGCLoopGain;
      | 
      | % CS parameters
      | CSKp                   = RxParams.CSKp;
      | CSK0                   = RxParams.CSK0;  
      | CSLoopFilterPropGain   = RxParams.CSLoopFilterPropGain;
      | CSLoopFilterIntegGain  = RxParams.CSLoopFilterIntegGain;
      | CFOChangeDetectThreshold = RxParams.CFOChangeDetectThreshold;
      | 
      | % SS parameters
      | SSKp                   = RxParams.SSKp; 
      | SSK0                   = RxParams.SSK0;  
      | SSLoopFilterPropGain   = RxParams.SSLoopFilterPropGain;
      | SSLoopFilterIntegGain  = RxParams.SSLoopFilterIntegGain;
      | 
      | % preamble detector parameters
      | searchSamples          = dataBits/2;
      | 
      | clear RxParams;
  QPSK Tx : Subsystem  mask{dataBits=size(cfg.frames,1)*8}
      mask prompts: dataBits "No. Data Bits in Frame"
      mask init:
      | TxParams            = zynqRadioHWSWQPSKTxRxParameters();
      | Preamble            = TxParams.Preamble;
      | QPSKConstellation   = TxParams.QPSKConstellation;
      | dataBitsPerPacket   = dataBits;
      | SamplesPerSymbol    = TxParams.SamplesPerSymbol;
      | RRCCoef             = TxParams.RRCCoef;
      | dataRAMAddrWidth    = nextpow2(dataBitsPerPacket*2)+5;
      | bitsPerPacket       = dataBitsPerPacket + length(Preamble);
      | 
      | clear TxParams;
  Switch : Switch  Criteria=u2 ~= 0  Threshold=1  SaturateOnIntegerOverflow=off  InputSameDT=off
  Switch3 : Switch  Criteria=u2 ~= 0  Threshold=1  SaturateOnIntegerOverflow=off  InputSameDT=off
  channel : Subsystem  Commented=on
  txDataOut : Outport
  txValidOut : Outport  Port=2
  rxDataOut : Outport  Port=3
  rxCtrlOut : Outport  Port=4
  rxDiagBus : Outport  Port=5
  channelDataOut : Outport  Port=6
  channelValidOut : Outport  Port=7
  wires:
  dataIn/1 -> QPSK Tx/1(dataIn)
  QPSK Rx/3(rxDiagBus) -> rxDiagBus/1
  QPSK Rx/1(dataOut) -> rxDataOut/1
  QPSK Rx/2(ctrlOut) -> rxCtrlOut/1
  Data Type Conversion7/1 -> QPSK Rx/1(dataIn)
  Switch3/1 -> QPSK Rx/2(validIn)
  validIn/1 -> QPSK Tx/2(validIn)
  Switch/1 -> Data Type Conversion7/1
  normalisedPhase/1 -> channel/4(normalisedPhase)
  normalisedFreq/1 -> channel/3(normalisedFreq)
  QPSK Tx/2(validOut) -> txValidOut/1, channel/2(validIn)
  QPSK Tx/1(dataOut) -> txDataOut/1, channel/1(dataIn)
  overAir/1 -> Switch3/2, Switch/2
  rstCS/1 -> QPSK Rx/3(rstCS)
  overAirDataIn/1 -> Switch/1
  overAirValidIn/1 -> Switch3/1
  channel/2(validOut) -> channelValidOut/1, Switch3/3
  channel/1(dataOut) -> channelDataOut/1, Switch/3
  chirpEn/1 -> channel/5(chirpEn)

== system frft_qpsk_transceiver/Model Parameters/HDL_QPSK/Subsystem ==
  bits : Inport
  bitsCtrl : Inport  Port=2
  rxBus : Inport  Port=3
  reset : Inport  Port=4
  BER : Subsystem
  Bit Concat : hdlsllib/Logic and Bit Operations/Bit Concat  numInputs=3
  Bits to Char : Subsystem
  Bus Selector1 : BusSelector  OutputSignals=startOut,validOut,endOut
  Bus Selector2 : BusSelector  OutputSignals=nSynced,QPSKConstellationValid,QPSKConstellationPoints,normCoarseFreqEst
  Bus Selector3 : BusSelector  Commented=on  OutputSignals=startOut,validOut,endOut
  Complex to Real-Imag : ComplexToRealImag
  DVB-S2 BCH Decoder : whdledac/DVB-S2 BCH Decoder  Commented=on  FECFrameSource=Property  FECFrameType=Short  CodeRateSource=Property  CodeRateNormal=1/4  CodeRateShort=1/4  NumErrorsOutputPort=on  SimulateUsing=Code generation
  DVB-S2 LDPC Decoder : whdledac/DVB-S2 LDPC Decoder  Commented=on  FECFrameSource=Property  FECFrame=Short  CodeRateSource=Property  CodeRateNormal=1/4  CodeRateShort=1/4  Parallelism=45  Algorithm=Min-sum  SourceScalingFactor=Property  ScalingFactor=0.75  Termination=Max  SpecifyInputs=Property  NumIterations=63  MaxNumIterations=nIter  ParityCheckStatus=off  SimulateUsing=Code generation
  Data Type Conversion : DataTypeConversion  Commented=on  OutMin=0  OutMax=1  OutDataTypeStr=int8  SaturateOnIntegerOverflow=off  RndMeth=Floor
  Data Type Conversion1 : DataTypeConversion  OutDataTypeStr=int16  ConvertRealWorld=Stored Integer (SI)  SaturateOnIntegerOverflow=off  RndMeth=Floor
  Data Type Conversion3 : DataTypeConversion  OutDataTypeStr=uint32  SaturateOnIntegerOverflow=off  RndMeth=Floor
  Delay : Delay  Commented=on  DelayLength=1
  HDL Counter : hdlsllib/Sources/HDL Counter  CountType=Free running  CountInit=0  CountStep=1  CountMax=25  CountFromType=Initial value  CountFrom=0  CountResetPort=on  CountLoadPort=off  CountEnbPort=on  CountDirPort=off  CountHitOutputPort=off  CountDataType=Unsigned  CountWordLen=32  CountFracLen=0  CountSampTime=1
  Sample Control Bus Creator1 : whdlutilities/Sample Control Bus Creator  Commented=on
  bitCount : Outport
  bitErrors : Outport  Port=2
  char : Outport  Port=3
  charValid : Outport  Port=4
  Out5 : Outport  Port=5
  Out6 : Outport  Port=6
  Out7 : Outport  Port=7
  Out8 : Outport  Port=8
  coarseFreq : Outport  Port=9
  wires:
  BER/2(bitErrors) -> bitErrors/1
  Bus Selector1/1 -> BER/2(resetcounter), Bits to Char/2(start)  "<startOut>"
  reset/1 -> HDL Counter/1, BER/3(reset)
  Complex to Real-Imag/2 -> Out8/1
  Bus Selector2/4 -> coarseFreq/1  "<normCoarseFreqEst>"
  Bus Selector2/1 -> HDL Counter/2  "<nSynced>"
  Complex to Real-Imag/1 -> Out6/1
  HDL Counter/1 -> Out7/1
  Bus Selector2/3 -> Data Type Conversion1/1  "<QPSKConstellationPoints>"
  Data Type Conversion3/1 -> char/1
  Bits to Char/4(charValid) -> charValid/1
  Data Type Conversion1/1 -> Complex to Real-Imag/1
  bits/1 -> Data Type Conversion/1, BER/4(userBits), Bits to Char/1(data)
  Bus Selector1/2 -> BER/1(userBitsValid), Bits to Char/3(valid)  "<validOut>"
  BER/1(bitCount) -> bitCount/1
  Bus Selector2/2 -> Out5/1  "<QPSKConstellationValid>"
  rxBus/1 -> Bus Selector2/1
  Bus Selector1/3 -> Bits to Char/4(end)  "<endOut>"
  Bit Concat/1 -> Data Type Conversion3/1
  Bits to Char/1(frmStartOut) -> Bit Concat/1
  Bits to Char/2(frmEndOut) -> Bit Concat/2
  Bits to Char/3(charOut) -> Bit Concat/3
  DVB-S2 LDPC Decoder/2 -> DVB-S2 BCH Decoder/2  "ldpc_ctrl"
  DVB-S2 LDPC Decoder/1 -> DVB-S2 BCH Decoder/1  "dataOut"
  DVB-S2 LDPC Decoder/3 -> ?  "ldpc_next"
  DVB-S2 BCH Decoder/1 -> ?  "bchDataOut"
  DVB-S2 BCH Decoder/2 -> ?  "bch_ctrl"
  DVB-S2 BCH Decoder/3 -> ?  "bch_corrected"
  DVB-S2 BCH Decoder/4 -> ?  "bch_next"
  Data Type Conversion/1 -> DVB-S2 LDPC Decoder/1
  bitsCtrl/1 -> Delay/1, Bus Selector1/1
  Bus Selector3/1 -> Sample Control Bus Creator1/1  "<startOut>"
  Bus Selector3/3 -> Sample Control Bus Creator1/2  "<endOut>"
  Bus Selector3/2 -> Sample Control Bus Creator1/3  "<validOut>"
  Delay/1 -> Bus Selector3/1
  Sample Control Bus Creator1/1 -> DVB-S2 LDPC Decoder/2
